simulink model "ph_zitai"  (Simulink 6.2)
settings: Solver=ode3  StartTime=0.0  StopTime=10  FixedStep=0.005  RelTol=1e-3
values from neighbouring files (symbols this model uses):
  b22 = 0    [sim_3dof.m]
  b24 = (ph2(ma_cnt,alpha_cnt)-ph1(ma_cnt,alpha_cnt))/(1/57.3)/jy*Q*serf*L    [sim_3dof.m]
  b34 = (Ft-(C2(ma_cnt,alpha_cnt)-C1(ma_cnt,alpha_cnt))/(1/57.3)*Q*serf)/(m*v)    [sim_3dof.m]
  km_h = [0.873387605804 0.909736736815]    [hengce.mat]
  t1_h = [-5.72286727263 -5.49461503945]    [hengce.mat]
  tm_h = [-0.365121120283 -0.348561137688]    [hengce.mat]
  zeta_h = [-0.00997234611163 -0.0099155259514]    [hengce.mat]
settings Model: LastModifiedBy=wangjsh
settings DebuggingCC: SolverPrmCheckMsg=warning

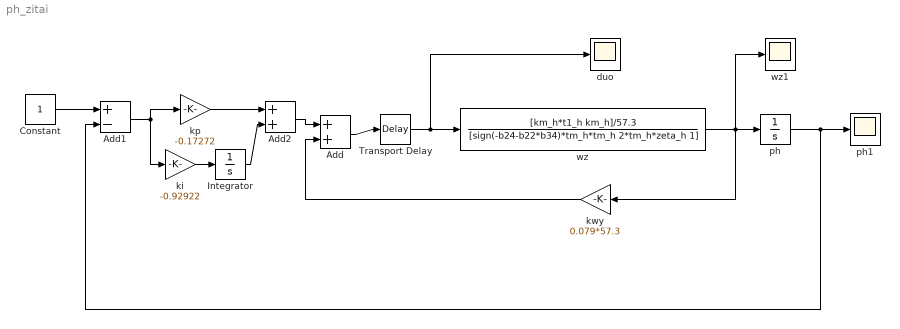
== system ph_zitai ==
  Add : Sum  OutScaling=2^-10
  Add1 : Sum  Inputs=+-  OutScaling=2^-10
  Add2 : Sum  OutScaling=2^-10
  Constant : Constant
  Integrator : Integrator
  Transport Delay : TransportDelay  DelayTime=0
  duo : Scope
      settings: SaveName=ScopeData2
  ki : Gain  Gain=-0.92922
  kp : Gain  Gain=-0.17272
  kwy : Gain  Orientation=left  Gain=0.079*57.3
  ph : Integrator
  ph1 : Scope
  wz : TransferFcn  Numerator=[km_h*t1_h km_h]/57.3  Denominator=[sign(-b24-b22*b34)*tm_h*tm_h 2*tm_h*zeta_h 1]
  wz1 : Scope
  wires:
  wz/1 -> ph/1, kwy/1, wz1/1
  Add/1 -> Transport Delay/1
  kwy/1 -> Add/2
  ph/1 -> ph1/1, Add1/2
  Constant/1 -> Add1/1
  Add2/1 -> Add/1
  Add1/1 -> kp/1, ki/1
  Integrator/1 -> Add2/2
  kp/1 -> Add2/1
  ki/1 -> Integrator/1
  Transport Delay/1 -> wz/1, duo/1
